simulink model "project"  (R2017b)
settings: Solver=FixedStepDiscrete  StartTime=0.0  StopTime=1  RelTol=1e-3
PreLoadFcn:
  | load('commwlan80211BusTypes')
PostLoadFcn:
  | commwlan80211BeaconModelParams('init')
InitFcn:
  | load('commwlan80211BusTypes')
model workspace: external: MAT-File (data not in the file)
undefined symbols (not defined in the file or in its folder): commwlan80211TxFilt, p80211
libraries: commutil2 x6, commwlan80211BeaconLib x6, commcrc2 x3, commchan3 x3, commrflib2 x3, commdigbbndpm3 x2, commsequence2 x2, commfilt2 x2, simulink x1, commsync2 x1, dspsigops x1, commblksprivate x1
(part 2 of 2)

== matlab function project/802.11 Transmitter/MAC Sublayer/Transmitter Controller ==
  settings: updateMethod=DISCRETE  sampleTime=p80211.MaximumPPDULength/p80211.SymbolRate
  data: payload output uint8 size=[p80211.MaximumMPDULength 1]; startTx output boolean; p80211 parameter
function [payload, startTx] = txCtrl(p80211)
%#codegen

persistent xmtState txOn mpduCount TSF

% States
Idle     = 0;
Transmit = 1;

% Initialize transmitter
if isempty(xmtState)
  TSF = zeros(2,1,'uint32');
  xmtState = Idle;
  txOn = false;
  mpduCount = p80211.BeaconInterval-1;
end

% Init payload buffer
[mpduHeader, mpduBody] = getBeaconMPDU(TSF, p80211);
payload = serializeMPDUData(mpduHeader, mpduBody);

% Update counter
mpduCount = mpduCount + 1;

% State machine
switch xmtState
  case Idle,
    if (mpduCount >= p80211.BeaconInterval)
      mpduCount = 0;
      [mpduHeader, mpduBody] = getBeaconMPDU(TSF, p80211);
      payload = serializeMPDUData(mpduHeader, mpduBody);
      txOn = true;
      xmtState = Transmit;
    end
  case Transmit,
      txOn = false;
      xmtState = Idle;
end

% Update TSF
oldTSF1 = TSF(1);
% Since bit rate is 1 Mbps, every bit is one microsecond.  Also, the
% transmitter works every (p80211.MaximumPPDULength = 1024) TU.
TSF(1) = TSF(1) + uint32(p80211.MaximumPPDULength); 
if oldTSF1 > TSF(1)
  TSF(2) = TSF(2) + 1;
end

% Update outputs
startTx = txOn;
end
